simulink model "test_liou"  (R2015b)
settings: Solver=VariableStepAuto  StartTime=0.0  StopTime=10.0  RelTol=1e-3
settings Model: Creator=think  LastModifiedBy=liuyuchen

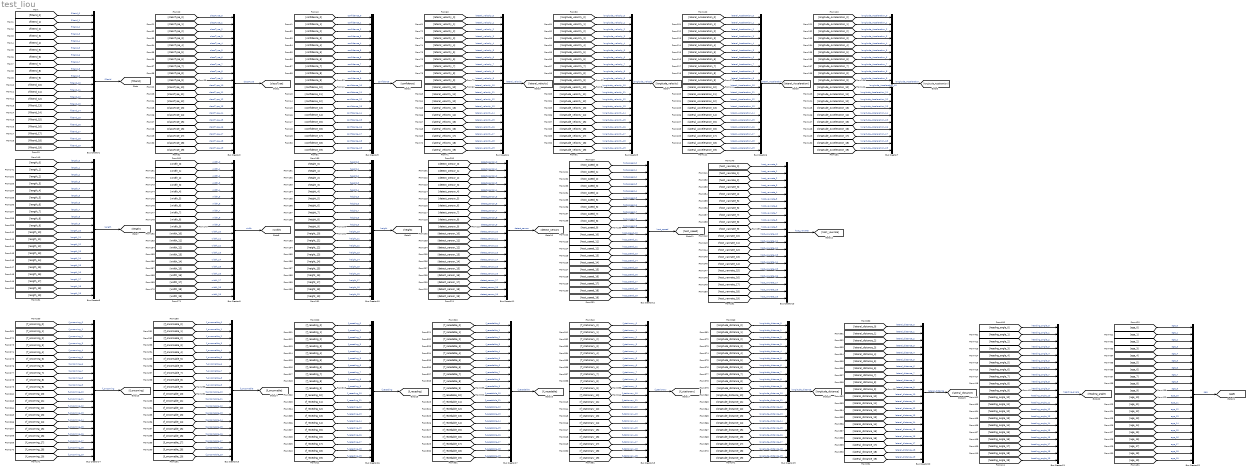
== system test_liou ==
  Bus Creator{1..22} (22 alike) : BusCreator  Inputs=20
  wires:
  [filterId_1] -> Bus Creator1/2  "filterId_1"
  [filterId_0] -> Bus Creator1/1  "filterId_0"
  [filterId_3] -> Bus Creator1/4  "filterId_3"
  [filterId_2] -> Bus Creator1/3  "filterId_2"
  [filterId_5] -> Bus Creator1/6  "filterId_5"
  [filterId_4] -> Bus Creator1/5  "filterId_4"
  [filterId_7] -> Bus Creator1/8  "filterId_7"
  [filterId_6] -> Bus Creator1/7  "filterId_6"
  [filterId_9] -> Bus Creator1/10  "filterId_9"
  [filterId_8] -> Bus Creator1/9  "filterId_8"
  [filterId_11] -> Bus Creator1/12  "filterId_11"
  [filterId_10] -> Bus Creator1/11  "filterId_10"
  [filterId_13] -> Bus Creator1/14  "filterId_13"
  [filterId_12] -> Bus Creator1/13  "filterId_12"
  [filterId_15] -> Bus Creator1/16  "filterId_15"
  [filterId_14] -> Bus Creator1/15  "filterId_14"
  [filterId_17] -> Bus Creator1/18  "filterId_17"
  [filterId_16] -> Bus Creator1/17  "filterId_16"
  [filterId_19] -> Bus Creator1/20  "filterId_19"
  [filterId_18] -> Bus Creator1/19  "filterId_18"
  Bus Creator1/1 -> [filterId]  "filterId"
  [classType_1] -> Bus Creator2/2  "classType_1"
  [classType_0] -> Bus Creator2/1  "classType_0"
  [classType_3] -> Bus Creator2/4  "classType_3"
  [classType_2] -> Bus Creator2/3  "classType_2"
  [classType_5] -> Bus Creator2/6  "classType_5"
  [classType_4] -> Bus Creator2/5  "classType_4"
  [classType_7] -> Bus Creator2/8  "classType_7"
  [classType_6] -> Bus Creator2/7  "classType_6"
  [classType_9] -> Bus Creator2/10  "classType_9"
  [classType_8] -> Bus Creator2/9  "classType_8"
  [classType_11] -> Bus Creator2/12  "classType_11"
  [classType_10] -> Bus Creator2/11  "classType_10"
  [classType_13] -> Bus Creator2/14  "classType_13"
  [classType_12] -> Bus Creator2/13  "classType_12"
  [classType_15] -> Bus Creator2/16  "classType_15"
  [classType_14] -> Bus Creator2/15  "classType_14"
  [classType_17] -> Bus Creator2/18  "classType_17"
  [classType_16] -> Bus Creator2/17  "classType_16"
  [classType_19] -> Bus Creator2/20  "classType_19"
  [classType_18] -> Bus Creator2/19  "classType_18"
  Bus Creator2/1 -> [classType]  "classType"
  [confidence_1] -> Bus Creator3/2  "confidence_1"
  [confidence_0] -> Bus Creator3/1  "confidence_0"
  [confidence_3] -> Bus Creator3/4  "confidence_3"
  [confidence_2] -> Bus Creator3/3  "confidence_2"
  [confidence_5] -> Bus Creator3/6  "confidence_5"
  [confidence_4] -> Bus Creator3/5  "confidence_4"
  [confidence_7] -> Bus Creator3/8  "confidence_7"
  [confidence_6] -> Bus Creator3/7  "confidence_6"
  [confidence_9] -> Bus Creator3/10  "confidence_9"
  [confidence_8] -> Bus Creator3/9  "confidence_8"
  [confidence_11] -> Bus Creator3/12  "confidence_11"
  [confidence_10] -> Bus Creator3/11  "confidence_10"
  [confidence_13] -> Bus Creator3/14  "confidence_13"
  [confidence_12] -> Bus Creator3/13  "confidence_12"
  [confidence_15] -> Bus Creator3/16  "confidence_15"
  [confidence_14] -> Bus Creator3/15  "confidence_14"
  [confidence_17] -> Bus Creator3/18  "confidence_17"
  [confidence_16] -> Bus Creator3/17  "confidence_16"
  [confidence_19] -> Bus Creator3/20  "confidence_19"
  [confidence_18] -> Bus Creator3/19  "confidence_18"
  Bus Creator3/1 -> [confidence]  "confidence"
  [lateral_velocity_1] -> Bus Creator4/2  "lateral_velocity_1"
  [lateral_velocity_0] -> Bus Creator4/1  "lateral_velocity_0"
  [lateral_velocity_3] -> Bus Creator4/4  "lateral_velocity_3"
  [lateral_velocity_2] -> Bus Creator4/3  "lateral_velocity_2"
  [lateral_velocity_5] -> Bus Creator4/6  "lateral_velocity_5"
  [lateral_velocity_4] -> Bus Creator4/5  "lateral_velocity_4"
  [lateral_velocity_7] -> Bus Creator4/8  "lateral_velocity_7"
  [lateral_velocity_6] -> Bus Creator4/7  "lateral_velocity_6"
  [lateral_velocity_9] -> Bus Creator4/10  "lateral_velocity_9"
  [lateral_velocity_8] -> Bus Creator4/9  "lateral_velocity_8"
  [lateral_velocity_11] -> Bus Creator4/12  "lateral_velocity_11"
  [lateral_velocity_10] -> Bus Creator4/11  "lateral_velocity_10"
  [lateral_velocity_13] -> Bus Creator4/14  "lateral_velocity_13"
  [lateral_velocity_12] -> Bus Creator4/13  "lateral_velocity_12"
  [lateral_velocity_15] -> Bus Creator4/16  "lateral_velocity_15"
  [lateral_velocity_14] -> Bus Creator4/15  "lateral_velocity_14"
  [lateral_velocity_17] -> Bus Creator4/18  "lateral_velocity_17"
  [lateral_velocity_16] -> Bus Creator4/17  "lateral_velocity_16"
  [lateral_velocity_19] -> Bus Creator4/20  "lateral_velocity_19"
  [lateral_velocity_18] -> Bus Creator4/19  "lateral_velocity_18"
  Bus Creator4/1 -> [lateral_velocity]  "lateral_velocity"
  [longitude_velocity_1] -> Bus Creator5/2  "longitude_velocity_1"
  [longitude_velocity_0] -> Bus Creator5/1  "longitude_velocity_0"
  [longitude_velocity_3] -> Bus Creator5/4  "longitude_velocity_3"
  [longitude_velocity_2] -> Bus Creator5/3  "longitude_velocity_2"
  [longitude_velocity_5] -> Bus Creator5/6  "longitude_velocity_5"
  [longitude_velocity_4] -> Bus Creator5/5  "longitude_velocity_4"
  [longitude_velocity_7] -> Bus Creator5/8  "longitude_velocity_7"
  [longitude_velocity_6] -> Bus Creator5/7  "longitude_velocity_6"
  [longitude_velocity_9] -> Bus Creator5/10  "longitude_velocity_9"
  [longitude_velocity_8] -> Bus Creator5/9  "longitude_velocity_8"
  [longitude_velocity_11] -> Bus Creator5/12  "longitude_velocity_11"
  [longitude_velocity_10] -> Bus Creator5/11  "longitude_velocity_10"
  [longitude_velocity_13] -> Bus Creator5/14  "longitude_velocity_13"
  [longitude_velocity_12] -> Bus Creator5/13  "longitude_velocity_12"
  [longitude_velocity_15] -> Bus Creator5/16  "longitude_velocity_15"
  [longitude_velocity_14] -> Bus Creator5/15  "longitude_velocity_14"
  [longitude_velocity_17] -> Bus Creator5/18  "longitude_velocity_17"
  [longitude_velocity_16] -> Bus Creator5/17  "longitude_velocity_16"
  [longitude_velocity_19] -> Bus Creator5/20  "longitude_velocity_19"
  [longitude_velocity_18] -> Bus Creator5/19  "longitude_velocity_18"
  Bus Creator5/1 -> [longitude_velocity]  "longitude_velocity"
  [lateral_Acceleration_1] -> Bus Creator6/2  "lateral_Acceleration_1"
  [lateral_Acceleration_0] -> Bus Creator6/1  "lateral_Acceleration_0"
  [lateral_Acceleration_3] -> Bus Creator6/4  "lateral_Acceleration_3"
  [lateral_Acceleration_2] -> Bus Creator6/3  "lateral_Acceleration_2"
  [lateral_Acceleration_5] -> Bus Creator6/6  "lateral_Acceleration_5"
  [lateral_Acceleration_4] -> Bus Creator6/5  "lateral_Acceleration_4"
  [lateral_Acceleration_7] -> Bus Creator6/8  "lateral_Acceleration_7"
  [lateral_Acceleration_6] -> Bus Creator6/7  "lateral_Acceleration_6"
  [lateral_Acceleration_9] -> Bus Creator6/10  "lateral_Acceleration_9"
  [lateral_Acceleration_8] -> Bus Creator6/9  "lateral_Acceleration_8"
  [lateral_Acceleration_11] -> Bus Creator6/12  "lateral_Acceleration_11"
  [lateral_Acceleration_10] -> Bus Creator6/11  "lateral_Acceleration_10"
  [lateral_Acceleration_13] -> Bus Creator6/14  "lateral_Acceleration_13"
  [lateral_Acceleration_12] -> Bus Creator6/13  "lateral_Acceleration_12"
  [lateral_Acceleration_15] -> Bus Creator6/16  "lateral_Acceleration_15"
  [lateral_Acceleration_14] -> Bus Creator6/15  "lateral_Acceleration_14"
  [lateral_Acceleration_17] -> Bus Creator6/18  "lateral_Acceleration_17"
  [lateral_Acceleration_16] -> Bus Creator6/17  "lateral_Acceleration_16"
  [lateral_Acceleration_19] -> Bus Creator6/20  "lateral_Acceleration_19"
  [lateral_Acceleration_18] -> Bus Creator6/19  "lateral_Acceleration_18"
  Bus Creator6/1 -> [lateral_Acceleration]  "lateral_Acceleration"
  [longitude_Acceleration_1] -> Bus Creator7/2  "longitude_Acceleration_1"
  [longitude_Acceleration_0] -> Bus Creator7/1  "longitude_Acceleration_0"
  [longitude_Acceleration_3] -> Bus Creator7/4  "longitude_Acceleration_3"
  [longitude_Acceleration_2] -> Bus Creator7/3  "longitude_Acceleration_2"
  [longitude_Acceleration_5] -> Bus Creator7/6  "longitude_Acceleration_5"
  [longitude_Acceleration_4] -> Bus Creator7/5  "longitude_Acceleration_4"
  [longitude_Acceleration_7] -> Bus Creator7/8  "longitude_Acceleration_7"
  [longitude_Acceleration_6] -> Bus Creator7/7  "longitude_Acceleration_6"
  [longitude_Acceleration_9] -> Bus Creator7/10  "longitude_Acceleration_9"
  [longitude_Acceleration_8] -> Bus Creator7/9  "longitude_Acceleration_8"
  [longitude_Acceleration_11] -> Bus Creator7/12  "longitude_Acceleration_11"
  [longitude_Acceleration_10] -> Bus Creator7/11  "longitude_Acceleration_10"
  [longitude_Acceleration_13] -> Bus Creator7/14  "longitude_Acceleration_13"
  [longitude_Acceleration_12] -> Bus Creator7/13  "longitude_Acceleration_12"
  [longitude_Acceleration_15] -> Bus Creator7/16  "longitude_Acceleration_15"
  [longitude_Acceleration_14] -> Bus Creator7/15  "longitude_Acceleration_14"
  [longitude_Acceleration_17] -> Bus Creator7/18  "longitude_Acceleration_17"
  [longitude_Acceleration_16] -> Bus Creator7/17  "longitude_Acceleration_16"
  [longitude_Acceleration_19] -> Bus Creator7/20  "longitude_Acceleration_19"
  [longitude_Acceleration_18] -> Bus Creator7/19  "longitude_Acceleration_18"
  Bus Creator7/1 -> [longitude_Acceleration]  "longitude_Acceleration"
  [length_1] -> Bus Creator8/2  "length_1"
  [length_0] -> Bus Creator8/1  "length_0"
  [length_3] -> Bus Creator8/4  "length_3"
  [length_2] -> Bus Creator8/3  "length_2"
  [length_5] -> Bus Creator8/6  "length_5"
  [length_4] -> Bus Creator8/5  "length_4"
  [length_7] -> Bus Creator8/8  "length_7"
  [length_6] -> Bus Creator8/7  "length_6"
  [length_9] -> Bus Creator8/10  "length_9"
  [length_8] -> Bus Creator8/9  "length_8"
  [length_11] -> Bus Creator8/12  "length_11"
  [length_10] -> Bus Creator8/11  "length_10"
  [length_13] -> Bus Creator8/14  "length_13"
  [length_12] -> Bus Creator8/13  "length_12"
  [length_15] -> Bus Creator8/16  "length_15"
  [length_14] -> Bus Creator8/15  "length_14"
  [length_17] -> Bus Creator8/18  "length_17"
  [length_16] -> Bus Creator8/17  "length_16"
  [length_19] -> Bus Creator8/20  "length_19"
  [length_18] -> Bus Creator8/19  "length_18"
  Bus Creator8/1 -> [length]  "length"
  [width_1] -> Bus Creator9/2  "width_1"
  [width_0] -> Bus Creator9/1  "width_0"
  [width_3] -> Bus Creator9/4  "width_3"
  [width_2] -> Bus Creator9/3  "width_2"
  [width_5] -> Bus Creator9/6  "width_5"
  [width_4] -> Bus Creator9/5  "width_4"
  [width_7] -> Bus Creator9/8  "width_7"
  [width_6] -> Bus Creator9/7  "width_6"
  [width_9] -> Bus Creator9/10  "width_9"
  [width_8] -> Bus Creator9/9  "width_8"
  [width_11] -> Bus Creator9/12  "width_11"
  [width_10] -> Bus Creator9/11  "width_10"
  [width_13] -> Bus Creator9/14  "width_13"
  [width_12] -> Bus Creator9/13  "width_12"
  [width_15] -> Bus Creator9/16  "width_15"
  [width_14] -> Bus Creator9/15  "width_14"
  [width_17] -> Bus Creator9/18  "width_17"
  [width_16] -> Bus Creator9/17  "width_16"
  [width_19] -> Bus Creator9/20  "width_19"
  [width_18] -> Bus Creator9/19  "width_18"
  Bus Creator9/1 -> [width]  "width"
  [height_1] -> Bus Creator10/2  "height_1"
  [height_0] -> Bus Creator10/1  "height_0"
  [height_3] -> Bus Creator10/4  "height_3"
  [height_2] -> Bus Creator10/3  "height_2"
  [height_5] -> Bus Creator10/6  "height_5"
  [height_4] -> Bus Creator10/5  "height_4"
  [height_7] -> Bus Creator10/8  "height_7"
  [height_6] -> Bus Creator10/7  "height_6"
  [height_9] -> Bus Creator10/10  "height_9"
  [height_8] -> Bus Creator10/9  "height_8"
  [height_11] -> Bus Creator10/12  "height_11"
  [height_10] -> Bus Creator10/11  "height_10"
  [height_13] -> Bus Creator10/14  "height_13"
  [height_12] -> Bus Creator10/13  "height_12"
  [height_15] -> Bus Creator10/16  "height_15"
  [height_14] -> Bus Creator10/15  "height_14"
  [height_17] -> Bus Creator10/18  "height_17"
  [height_16] -> Bus Creator10/17  "height_16"
  [height_19] -> Bus Creator10/20  "height_19"
  [height_18] -> Bus Creator10/19  "height_18"
  Bus Creator10/1 -> [height]  "height"
  [detect_sensor_1] -> Bus Creator11/2  "detect_sensor_1"
  [detect_sensor_0] -> Bus Creator11/1  "detect_sensor_0"
  [detect_sensor_3] -> Bus Creator11/4  "detect_sensor_3"
  [detect_sensor_2] -> Bus Creator11/3  "detect_sensor_2"
  [detect_sensor_5] -> Bus Creator11/6  "detect_sensor_5"
  [detect_sensor_4] -> Bus Creator11/5  "detect_sensor_4"
  [detect_sensor_7] -> Bus Creator11/8  "detect_sensor_7"
  [detect_sensor_6] -> Bus Creator11/7  "detect_sensor_6"
  [detect_sensor_9] -> Bus Creator11/10  "detect_sensor_9"
  [detect_sensor_8] -> Bus Creator11/9  "detect_sensor_8"
  [detect_sensor_11] -> Bus Creator11/12  "detect_sensor_11"
  [detect_sensor_10] -> Bus Creator11/11  "detect_sensor_10"
  [detect_sensor_13] -> Bus Creator11/14  "detect_sensor_13"
  [detect_sensor_12] -> Bus Creator11/13  "detect_sensor_12"
  [detect_sensor_15] -> Bus Creator11/16  "detect_sensor_15"
  [detect_sensor_14] -> Bus Creator11/15  "detect_sensor_14"
  [detect_sensor_17] -> Bus Creator11/18  "detect_sensor_17"
  [detect_sensor_16] -> Bus Creator11/17  "detect_sensor_16"
  [detect_sensor_19] -> Bus Creator11/20  "detect_sensor_19"
  [detect_sensor_18] -> Bus Creator11/19  "detect_sensor_18"
  Bus Creator11/1 -> [detect_sensor]  "detect_sensor"
  [host_speed_1] -> Bus Creator12/2  "host_speed_1"
  [host_speed_0] -> Bus Creator12/1  "host_speed_0"
  [host_speed_3] -> Bus Creator12/4  "host_speed_3"
  [host_speed_2] -> Bus Creator12/3  "host_speed_2"
  [host_speed_5] -> Bus Creator12/6  "host_speed_5"
  [host_speed_4] -> Bus Creator12/5  "host_speed_4"
  [host_speed_7] -> Bus Creator12/8  "host_speed_7"
  [host_speed_6] -> Bus Creator12/7  "host_speed_6"
  [host_speed_9] -> Bus Creator12/10  "host_speed_9"
  [host_speed_8] -> Bus Creator12/9  "host_speed_8"
  [host_speed_11] -> Bus Creator12/12  "host_speed_11"
  [host_speed_10] -> Bus Creator12/11  "host_speed_10"
  [host_speed_13] -> Bus Creator12/14  "host_speed_13"
  [host_speed_12] -> Bus Creator12/13  "host_speed_12"
  [host_speed_15] -> Bus Creator12/16  "host_speed_15"
  [host_speed_14] -> Bus Creator12/15  "host_speed_14"
  [host_speed_17] -> Bus Creator12/18  "host_speed_17"
  [host_speed_16] -> Bus Creator12/17  "host_speed_16"
  [host_speed_19] -> Bus Creator12/20  "host_speed_19"
  [host_speed_18] -> Bus Creator12/19  "host_speed_18"
  Bus Creator12/1 -> [host_speed]  "host_speed"
  [host_yawrate_1] -> Bus Creator13/2  "host_yawrate_1"
  [host_yawrate_0] -> Bus Creator13/1  "host_yawrate_0"
  [host_yawrate_3] -> Bus Creator13/4  "host_yawrate_3"
  [host_yawrate_2] -> Bus Creator13/3  "host_yawrate_2"
  [host_yawrate_5] -> Bus Creator13/6  "host_yawrate_5"
  [host_yawrate_4] -> Bus Creator13/5  "host_yawrate_4"
  [host_yawrate_7] -> Bus Creator13/8  "host_yawrate_7"
  [host_yawrate_6] -> Bus Creator13/7  "host_yawrate_6"
  [host_yawrate_9] -> Bus Creator13/10  "host_yawrate_9"
  [host_yawrate_8] -> Bus Creator13/9  "host_yawrate_8"
  [host_yawrate_11] -> Bus Creator13/12  "host_yawrate_11"
  [host_yawrate_10] -> Bus Creator13/11  "host_yawrate_10"
  [host_yawrate_13] -> Bus Creator13/14  "host_yawrate_13"
  [host_yawrate_12] -> Bus Creator13/13  "host_yawrate_12"
  [host_yawrate_15] -> Bus Creator13/16  "host_yawrate_15"
  [host_yawrate_14] -> Bus Creator13/15  "host_yawrate_14"
  [host_yawrate_17] -> Bus Creator13/18  "host_yawrate_17"
  [host_yawrate_16] -> Bus Creator13/17  "host_yawrate_16"
  [host_yawrate_19] -> Bus Creator13/20  "host_yawrate_19"
  [host_yawrate_18] -> Bus Creator13/19  "host_yawrate_18"
  Bus Creator13/1 -> [host_yawrate]  "host_yawrate"
  [f_oncoming_1] -> Bus Creator14/2  "f_oncoming_1"
  [f_oncoming_0] -> Bus Creator14/1  "f_oncoming_0"
  [f_oncoming_3] -> Bus Creator14/4  "f_oncoming_3"
  [f_oncoming_2] -> Bus Creator14/3  "f_oncoming_2"
  [f_oncoming_5] -> Bus Creator14/6  "f_oncoming_5"
  [f_oncoming_4] -> Bus Creator14/5  "f_oncoming_4"
  [f_oncoming_7] -> Bus Creator14/8  "f_oncoming_7"
  [f_oncoming_6] -> Bus Creator14/7  "f_oncoming_6"
  [f_oncoming_9] -> Bus Creator14/10  "f_oncoming_9"
  [f_oncoming_8] -> Bus Creator14/9  "f_oncoming_8"
  [f_oncoming_11] -> Bus Creator14/12  "f_oncoming_11"
  [f_oncoming_10] -> Bus Creator14/11  "f_oncoming_10"
  [f_oncoming_13] -> Bus Creator14/14  "f_oncoming_13"
  [f_oncoming_12] -> Bus Creator14/13  "f_oncoming_12"
  [f_oncoming_15] -> Bus Creator14/16  "f_oncoming_15"
  [f_oncoming_14] -> Bus Creator14/15  "f_oncoming_14"
  [f_oncoming_17] -> Bus Creator14/18  "f_oncoming_17"
  [f_oncoming_16] -> Bus Creator14/17  "f_oncoming_16"
  [f_oncoming_19] -> Bus Creator14/20  "f_oncoming_19"
  [f_oncoming_18] -> Bus Creator14/19  "f_oncoming_18"
  Bus Creator14/1 -> [f_oncoming]  "f_oncoming"
  [f_oncomable_1] -> Bus Creator15/2  "f_oncomable_1"
  [f_oncomable_0] -> Bus Creator15/1  "f_oncomable_0"
  [f_oncomable_3] -> Bus Creator15/4  "f_oncomable_3"
  [f_oncomable_2] -> Bus Creator15/3  "f_oncomable_2"
  [f_oncomable_5] -> Bus Creator15/6  "f_oncomable_5"
  [f_oncomable_4] -> Bus Creator15/5  "f_oncomable_4"
  [f_oncomable_7] -> Bus Creator15/8  "f_oncomable_7"
  [f_oncomable_6] -> Bus Creator15/7  "f_oncomable_6"
  [f_oncomable_9] -> Bus Creator15/10  "f_oncomable_9"
  [f_oncomable_8] -> Bus Creator15/9  "f_oncomable_8"
  [f_oncomable_11] -> Bus Creator15/12  "f_oncomable_11"
  [f_oncomable_10] -> Bus Creator15/11  "f_oncomable_10"
  [f_oncomable_13] -> Bus Creator15/14  "f_oncomable_13"
  [f_oncomable_12] -> Bus Creator15/13  "f_oncomable_12"
  [f_oncomable_15] -> Bus Creator15/16  "f_oncomable_15"
  [f_oncomable_14] -> Bus Creator15/15  "f_oncomable_14"
  [f_oncomable_17] -> Bus Creator15/18  "f_oncomable_17"
  [f_oncomable_16] -> Bus Creator15/17  "f_oncomable_16"
  [f_oncomable_19] -> Bus Creator15/20  "f_oncomable_19"
  [f_oncomable_18] -> Bus Creator15/19  "f_oncomable_18"
  Bus Creator15/1 -> [f_oncomable]  "f_oncomable"
  [f_receding_1] -> Bus Creator16/2  "f_receding_1"
  [f_receding_0] -> Bus Creator16/1  "f_receding_0"
  [f_receding_3] -> Bus Creator16/4  "f_receding_3"
  [f_receding_2] -> Bus Creator16/3  "f_receding_2"
  [f_receding_5] -> Bus Creator16/6  "f_receding_5"
  [f_receding_4] -> Bus Creator16/5  "f_receding_4"
  [f_receding_7] -> Bus Creator16/8  "f_receding_7"
  [f_receding_6] -> Bus Creator16/7  "f_receding_6"
  [f_receding_9] -> Bus Creator16/10  "f_receding_9"
  [f_receding_8] -> Bus Creator16/9  "f_receding_8"
  [f_receding_11] -> Bus Creator16/12  "f_receding_11"
  [f_receding_10] -> Bus Creator16/11  "f_receding_10"
  [f_receding_13] -> Bus Creator16/14  "f_receding_13"
  [f_receding_12] -> Bus Creator16/13  "f_receding_12"
  [f_receding_15] -> Bus Creator16/16  "f_receding_15"
  [f_receding_14] -> Bus Creator16/15  "f_receding_14"
  [f_receding_17] -> Bus Creator16/18  "f_receding_17"
  [f_receding_16] -> Bus Creator16/17  "f_receding_16"
  [f_receding_19] -> Bus Creator16/20  "f_receding_19"
  [f_receding_18] -> Bus Creator16/19  "f_receding_18"
  Bus Creator16/1 -> [f_receding]  "f_receding"
  [f_recedable_1] -> Bus Creator17/2  "f_recedable_1"
  [f_recedable_0] -> Bus Creator17/1  "f_recedable_0"
  [f_recedable_3] -> Bus Creator17/4  "f_recedable_3"
  [f_recedable_2] -> Bus Creator17/3  "f_recedable_2"
  [f_recedable_5] -> Bus Creator17/6  "f_recedable_5"
  [f_recedable_4] -> Bus Creator17/5  "f_recedable_4"
  [f_recedable_7] -> Bus Creator17/8  "f_recedable_7"
  [f_recedable_6] -> Bus Creator17/7  "f_recedable_6"
  [f_recedable_9] -> Bus Creator17/10  "f_recedable_9"
  [f_recedable_8] -> Bus Creator17/9  "f_recedable_8"
  [f_recedable_11] -> Bus Creator17/12  "f_recedable_11"
  [f_recedable_10] -> Bus Creator17/11  "f_recedable_10"
  [f_recedable_13] -> Bus Creator17/14  "f_recedable_13"
  [f_recedable_12] -> Bus Creator17/13  "f_recedable_12"
  [f_recedable_15] -> Bus Creator17/16  "f_recedable_15"
  [f_recedable_14] -> Bus Creator17/15  "f_recedable_14"
  [f_recedable_17] -> Bus Creator17/18  "f_recedable_17"
  [f_recedable_16] -> Bus Creator17/17  "f_recedable_16"
  [f_recedable_19] -> Bus Creator17/20  "f_recedable_19"
  [f_recedable_18] -> Bus Creator17/19  "f_recedable_18"
  Bus Creator17/1 -> [f_recedable]  "f_recedable"
  [f_stationary_1] -> Bus Creator18/2  "f_stationary_1"
  [f_stationary_0] -> Bus Creator18/1  "f_stationary_0"
  [f_stationary_3] -> Bus Creator18/4  "f_stationary_3"
  [f_stationary_2] -> Bus Creator18/3  "f_stationary_2"
  [f_stationary_5] -> Bus Creator18/6  "f_stationary_5"
  [f_stationary_4] -> Bus Creator18/5  "f_stationary_4"
  [f_stationary_7] -> Bus Creator18/8  "f_stationary_7"
  [f_stationary_6] -> Bus Creator18/7  "f_stationary_6"
  [f_stationary_9] -> Bus Creator18/10  "f_stationary_9"
  [f_stationary_8] -> Bus Creator18/9  "f_stationary_8"
  [f_stationary_11] -> Bus Creator18/12  "f_stationary_11"
  [f_stationary_10] -> Bus Creator18/11  "f_stationary_10"
  [f_stationary_13] -> Bus Creator18/14  "f_stationary_13"
  [f_stationary_12] -> Bus Creator18/13  "f_stationary_12"
  [f_stationary_15] -> Bus Creator18/16  "f_stationary_15"
  [f_stationary_14] -> Bus Creator18/15  "f_stationary_14"
  [f_stationary_17] -> Bus Creator18/18  "f_stationary_17"
  [f_stationary_16] -> Bus Creator18/17  "f_stationary_16"
  [f_stationary_19] -> Bus Creator18/20  "f_stationary_19"
  [f_stationary_18] -> Bus Creator18/19  "f_stationary_18"
  Bus Creator18/1 -> [f_stationary]  "f_stationary"
  [longitude_distance_1] -> Bus Creator19/2  "longitude_distance_1"
  [longitude_distance_0] -> Bus Creator19/1  "longitude_distance_0"
  [longitude_distance_3] -> Bus Creator19/4  "longitude_distance_3"
  [longitude_distance_2] -> Bus Creator19/3  "longitude_distance_2"
  [longitude_distance_5] -> Bus Creator19/6  "longitude_distance_5"
  [longitude_distance_4] -> Bus Creator19/5  "longitude_distance_4"
  [longitude_distance_7] -> Bus Creator19/8  "longitude_distance_7"
  [longitude_distance_6] -> Bus Creator19/7  "longitude_distance_6"
  [longitude_distance_9] -> Bus Creator19/10  "longitude_distance_9"
  [longitude_distance_8] -> Bus Creator19/9  "longitude_distance_8"
  [longitude_distance_11] -> Bus Creator19/12  "longitude_distance_11"
  [longitude_distance_10] -> Bus Creator19/11  "longitude_distance_10"
  [longitude_distance_13] -> Bus Creator19/14  "longitude_distance_13"
  [longitude_distance_12] -> Bus Creator19/13  "longitude_distance_12"
  [longitude_distance_15] -> Bus Creator19/16  "longitude_distance_15"
  [longitude_distance_14] -> Bus Creator19/15  "longitude_distance_14"
  [longitude_distance_17] -> Bus Creator19/18  "longitude_distance_17"
  [longitude_distance_16] -> Bus Creator19/17  "longitude_distance_16"
  [longitude_distance_19] -> Bus Creator19/20  "longitude_distance_19"
  [longitude_distance_18] -> Bus Creator19/19  "longitude_distance_18"
  Bus Creator19/1 -> [longitude_distance]  "longitude_distance"
  [lateral_distance_1] -> Bus Creator20/2  "lateral_distance_1"
  [lateral_distance_0] -> Bus Creator20/1  "lateral_distance_0"
  [lateral_distance_3] -> Bus Creator20/4  "lateral_distance_3"
  [lateral_distance_2] -> Bus Creator20/3  "lateral_distance_2"
  [lateral_distance_5] -> Bus Creator20/6  "lateral_distance_5"
  [lateral_distance_4] -> Bus Creator20/5  "lateral_distance_4"
  [lateral_distance_7] -> Bus Creator20/8  "lateral_distance_7"
  [lateral_distance_6] -> Bus Creator20/7  "lateral_distance_6"
  [lateral_distance_9] -> Bus Creator20/10  "lateral_distance_9"
  [lateral_distance_8] -> Bus Creator20/9  "lateral_distance_8"
  [lateral_distance_11] -> Bus Creator20/12  "lateral_distance_11"
  [lateral_distance_10] -> Bus Creator20/11  "lateral_distance_10"
  [lateral_distance_13] -> Bus Creator20/14  "lateral_distance_13"
  [lateral_distance_12] -> Bus Creator20/13  "lateral_distance_12"
  [lateral_distance_15] -> Bus Creator20/16  "lateral_distance_15"
  [lateral_distance_14] -> Bus Creator20/15  "lateral_distance_14"
  [lateral_distance_17] -> Bus Creator20/18  "lateral_distance_17"
  [lateral_distance_16] -> Bus Creator20/17  "lateral_distance_16"
  [lateral_distance_19] -> Bus Creator20/20  "lateral_distance_19"
  [lateral_distance_18] -> Bus Creator20/19  "lateral_distance_18"
  Bus Creator20/1 -> [lateral_distance]  "lateral_distance"
  [heading_angle_1] -> Bus Creator21/2  "heading_angle_1"
  [heading_angle_0] -> Bus Creator21/1  "heading_angle_0"
  [heading_angle_3] -> Bus Creator21/4  "heading_angle_3"
  [heading_angle_2] -> Bus Creator21/3  "heading_angle_2"
  [heading_angle_5] -> Bus Creator21/6  "heading_angle_5"
  [heading_angle_4] -> Bus Creator21/5  "heading_angle_4"
  [heading_angle_7] -> Bus Creator21/8  "heading_angle_7"
  [heading_angle_6] -> Bus Creator21/7  "heading_angle_6"
  [heading_angle_9] -> Bus Creator21/10  "heading_angle_9"
  [heading_angle_8] -> Bus Creator21/9  "heading_angle_8"
  [heading_angle_11] -> Bus Creator21/12  "heading_angle_11"
  [heading_angle_10] -> Bus Creator21/11  "heading_angle_10"
  [heading_angle_13] -> Bus Creator21/14  "heading_angle_13"
  [heading_angle_12] -> Bus Creator21/13  "heading_angle_12"
  [heading_angle_15] -> Bus Creator21/16  "heading_angle_15"
  [heading_angle_14] -> Bus Creator21/15  "heading_angle_14"
  [heading_angle_17] -> Bus Creator21/18  "heading_angle_17"
  [heading_angle_16] -> Bus Creator21/17  "heading_angle_16"
  [heading_angle_19] -> Bus Creator21/20  "heading_angle_19"
  [heading_angle_18] -> Bus Creator21/19  "heading_angle_18"
  Bus Creator21/1 -> [heading_angle]  "heading_angle"
  [age_1] -> Bus Creator22/2  "age_1"
  [age_0] -> Bus Creator22/1  "age_0"
  [age_3] -> Bus Creator22/4  "age_3"
  [age_2] -> Bus Creator22/3  "age_2"
  [age_5] -> Bus Creator22/6  "age_5"
  [age_4] -> Bus Creator22/5  "age_4"
  [age_7] -> Bus Creator22/8  "age_7"
  [age_6] -> Bus Creator22/7  "age_6"
  [age_9] -> Bus Creator22/10  "age_9"
  [age_8] -> Bus Creator22/9  "age_8"
  [age_11] -> Bus Creator22/12  "age_11"
  [age_10] -> Bus Creator22/11  "age_10"
  [age_13] -> Bus Creator22/14  "age_13"
  [age_12] -> Bus Creator22/13  "age_12"
  [age_15] -> Bus Creator22/16  "age_15"
  [age_14] -> Bus Creator22/15  "age_14"
  [age_17] -> Bus Creator22/18  "age_17"
  [age_16] -> Bus Creator22/17  "age_16"
  [age_19] -> Bus Creator22/20  "age_19"
  [age_18] -> Bus Creator22/19  "age_18"
  Bus Creator22/1 -> [age]  "age"
